simulink model "MyRhoVar"  (Simulink 7.9)
settings: Solver=FixedStepDiscrete  StartTime=0.0  StopTime=1e8  FixedStep=1  RelTol=1e-3
(part 3 of 3)

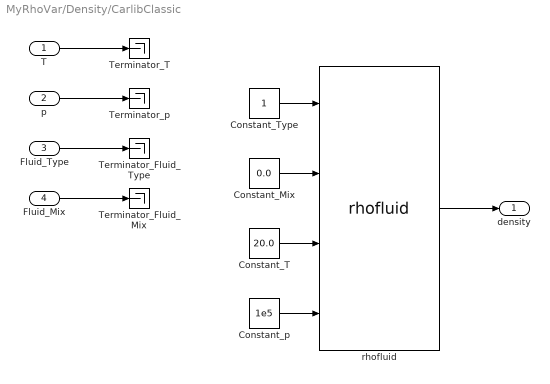
== system MyRhoVar/Density/CarlibClassic ==
  T : Inport
  p : Inport  Port=2
  Fluid_Type : Inport  Port=3
  Fluid_Mix : Inport  Port=4
  Constant_Mix : Constant  Value=0.0
  Constant_T : Constant  Value=20.0
  Constant_Type : Constant
  Constant_p : Constant  Value=1e5
  Terminator_Fluid_Mix : Terminator
  Terminator_Fluid_Type : Terminator
  Terminator_T : Terminator
  Terminator_p : Terminator
  rhofluid : S-Function  FunctionName=rhofluid  EnableBusSupport=off
  density : Outport
  wires:
  rhofluid/1 -> density/1
  T/1 -> Terminator_T/1
  p/1 -> Terminator_p/1
  Fluid_Type/1 -> Terminator_Fluid_Type/1
  Fluid_Mix/1 -> Terminator_Fluid_Mix/1
  Constant_T/1 -> rhofluid/3
  Constant_p/1 -> rhofluid/4
  Constant_Type/1 -> rhofluid/1
  Constant_Mix/1 -> rhofluid/2

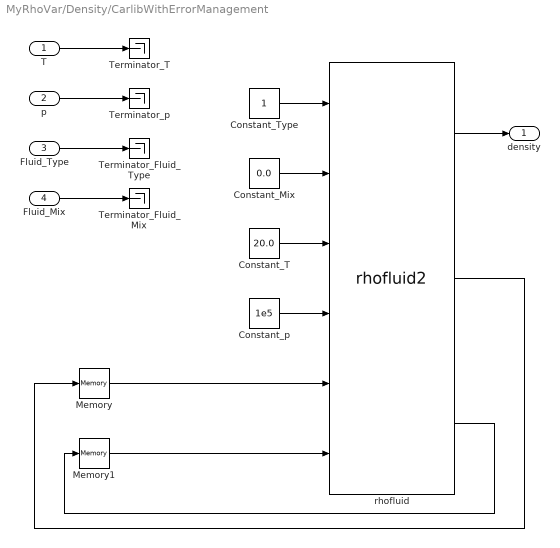
== system MyRhoVar/Density/CarlibWithErrorManagement ==
  T : Inport
  p : Inport  Port=2
  Fluid_Type : Inport  Port=3
  Fluid_Mix : Inport  Port=4
  Constant_Mix : Constant  Value=0.0
  Constant_T : Constant  Value=20.0
  Constant_Type : Constant
  Constant_p : Constant  Value=1e5
  Memory : Memory
  Memory1 : Memory
  Terminator_Fluid_Mix : Terminator
  Terminator_Fluid_Type : Terminator
  Terminator_T : Terminator
  Terminator_p : Terminator
  rhofluid : S-Function  FunctionName=rhofluid2  Parameters=DEBUGLEVEL-1,MAXTOTALWARNINGS,MAXCONSECUTIVEWARNINGS,WRITETOFILE,FILENAME  EnableBusSupport=off
  density : Outport
  wires:
  rhofluid/1 -> density/1
  rhofluid/2 -> Memory/1
  rhofluid/3 -> Memory1/1
  Memory1/1 -> rhofluid/6
  Memory/1 -> rhofluid/5
  T/1 -> Terminator_T/1
  p/1 -> Terminator_p/1
  Fluid_Type/1 -> Terminator_Fluid_Type/1
  Fluid_Mix/1 -> Terminator_Fluid_Mix/1
  Constant_T/1 -> rhofluid/3
  Constant_p/1 -> rhofluid/4
  Constant_Type/1 -> rhofluid/1
  Constant_Mix/1 -> rhofluid/2

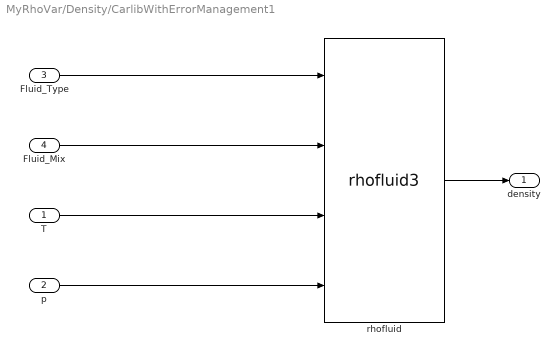
== system MyRhoVar/Density/CarlibWithErrorManagement1 ==
  T : Inport
  p : Inport  Port=2
  Fluid_Type : Inport  Port=3
  Fluid_Mix : Inport  Port=4
  rhofluid : S-Function  FunctionName=rhofluid3  Parameters=DEBUGLEVEL-1,MAXTOTALWARNINGS,MAXCONSECUTIVEWARNINGS,WRITETOFILE,FILENAME  EnableBusSupport=off
  density : Outport
  wires:
  rhofluid/1 -> density/1
  T/1 -> rhofluid/3
  p/1 -> rhofluid/4
  Fluid_Type/1 -> rhofluid/1
  Fluid_Mix/1 -> rhofluid/2

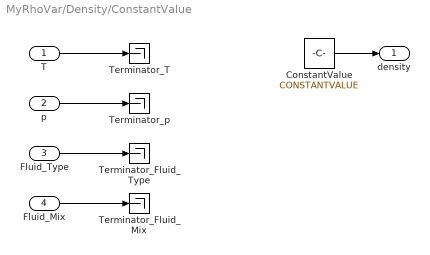
== system MyRhoVar/Density/ConstantValue ==
  T : Inport
  p : Inport  Port=2
  Fluid_Type : Inport  Port=3
  Fluid_Mix : Inport  Port=4
  ConstantValue : Constant  Value=CONSTANTVALUE
  Terminator_Fluid_Mix : Terminator
  Terminator_Fluid_Type : Terminator
  Terminator_T : Terminator
  Terminator_p : Terminator
  density : Outport
  wires:
  ConstantValue/1 -> density/1
  T/1 -> Terminator_T/1
  p/1 -> Terminator_p/1
  Fluid_Type/1 -> Terminator_Fluid_Type/1
  Fluid_Mix/1 -> Terminator_Fluid_Mix/1

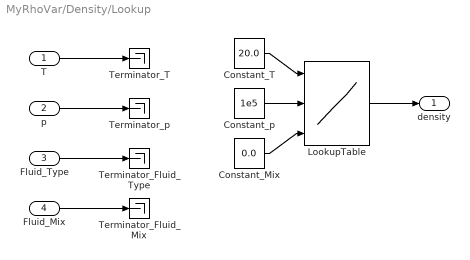
== system MyRhoVar/Density/Lookup ==
  T : Inport
  p : Inport  Port=2
  Fluid_Type : Inport  Port=3
  Fluid_Mix : Inport  Port=4
  Constant_Mix : Constant  Value=0.0
  Constant_T : Constant  Value=20.0
  Constant_p : Constant  Value=1e5
  LookupTable : Lookup_n-D  NumberOfTableDimensions=3  BreakpointsForDimension1=TLOOKUP  BreakpointsForDimension2=PLOOKUP  BreakpointsForDimension3=MIXLOOKUP  Table=DENSITYLOOKUP  DiagnosticForOutOfRangeInput=Warning  RndMeth=Simplest  InputSameDT=on
  Terminator_Fluid_Mix : Terminator
  Terminator_Fluid_Type : Terminator
  Terminator_T : Terminator
  Terminator_p : Terminator
  density : Outport
  wires:
  LookupTable/1 -> density/1
  T/1 -> Terminator_T/1
  p/1 -> Terminator_p/1
  Fluid_Type/1 -> Terminator_Fluid_Type/1
  Fluid_Mix/1 -> Terminator_Fluid_Mix/1
  Constant_T/1 -> LookupTable/1
  Constant_p/1 -> LookupTable/2
  Constant_Mix/1 -> LookupTable/3

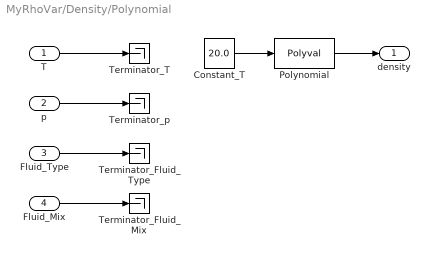
== system MyRhoVar/Density/Polynomial ==
  T : Inport
  p : Inport  Port=2
  Fluid_Type : Inport  Port=3
  Fluid_Mix : Inport  Port=4
  Constant_T : Constant  Value=20.0
  Polynomial : Polyval  Coefs=POLYNOMIALCOEFFICIENTS
  Terminator_Fluid_Mix : Terminator
  Terminator_Fluid_Type : Terminator
  Terminator_T : Terminator
  Terminator_p : Terminator
  density : Outport
  wires:
  Polynomial/1 -> density/1
  T/1 -> Terminator_T/1
  p/1 -> Terminator_p/1
  Fluid_Type/1 -> Terminator_Fluid_Type/1
  Fluid_Mix/1 -> Terminator_Fluid_Mix/1
  Constant_T/1 -> Polynomial/1
